simulink model "TV_Schema"  (R2024b)
settings: Solver=VariableStepAuto  StartTime=0.0  StopTime=3  RelTol=1e-3
model workspace (MAT data in the model file):
  Cyf = 60000
  Cyr = 60000
  Izz = 3000
  lf = 1.2
  lr = 1.5
  m = 1500
  tf = 0.65
  vx0 = 20
libraries: slpidlib x1
settings Model: Creator=junhyeongdoh  LastModifiedBy=junhyeongdoh

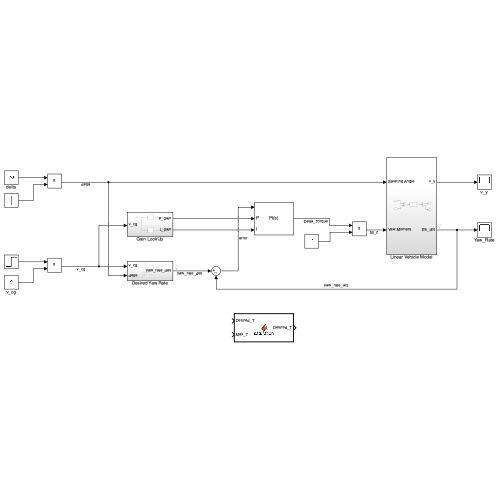
[thumbnail: Simulink's stored preview of the top-level diagram]
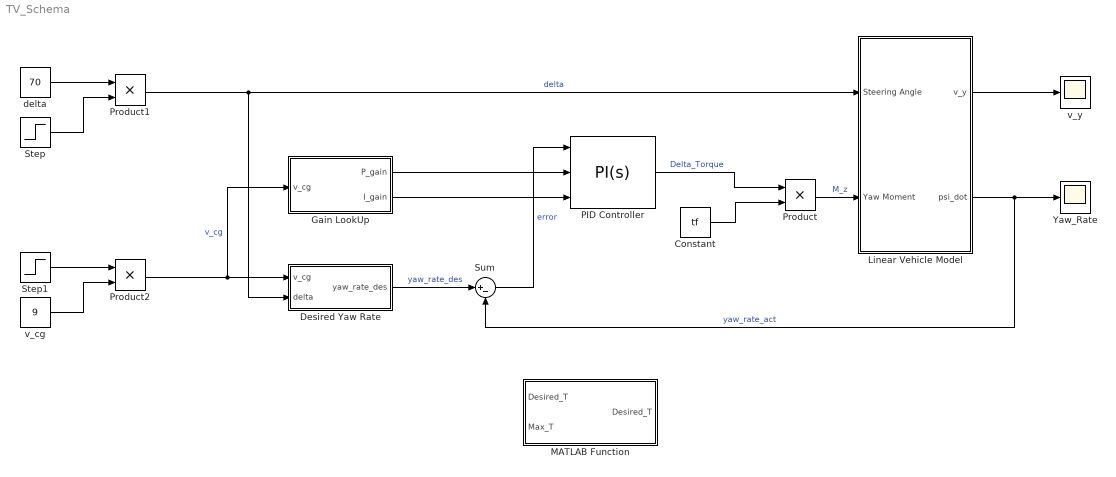
== system TV_Schema ==
  Constant : Constant  Value=tf
  Desired Yaw Rate : Subsystem
  Gain LookUp : Subsystem
  Linear Vehicle Model : Subsystem
  MATLAB Function : MATLAB Function  TreatAsAtomicUnit=on
  PID Controller : slpidlib/PID Controller  Controller=PI  Form=Parallel  TimeDomain=Continuous-time  UseExternalTs=off  SampleTime=-1  IntegratorMethod=Forward Euler  FilterMethod=Forward Euler  ControllerParametersSource=external  P=1  I=1  UseKiTs=off  D=0  UseExternalDerivativeSource=off  N=100  UseFilter=on  TunerSelectOption=Transfer Function Based (PID Tuner App)  InitialConditionSource=internal  InitialConditionForIntegrator=0  InitialConditionForFilter=0  DifferentiatorICPrevScaledInput=0  ExternalReset=none  TrackingMode=off  Kt=1  LimitOutput=off  SatLimitsSource=internal  UpperSaturationLimit=inf  LowerSaturationLimit=-inf  LinearizeAsGain=on  AntiWindupMode=none  Kb=1  LimitIntegrator=off  UpperIntegratorSaturationLimit=inf  LowerIntegratorSaturationLimit=-inf  POutMin=[]  POutMax=[]  IOutMin=[]  IOutMax=[]  DOutMin=[]  DOutMax=[]  NOutMin=[]  NOutMax=[]  SumOutMin=[]  SumOutMax=[]  SaturationOutMin=[]  SaturationOutMax=[]  PParamMin=[]  PParamMax=[]  IParamMin=[]  IParamMax=[]  DParamMin=[]  DParamMax=[]  NParamMin=[]  NParamMax=[]  KbParamMin=[]  KbParamMax=[]  KtParamMin=[]  KtParamMax=[]  KbOutMin=[]  KbOutMax=[]  KtOutMin=[]  KtOutMax=[]  IntegratorOutMin=[]  IntegratorOutMax=[]  FilterOutMin=[]  FilterOutMax=[]  SumI1OutMin=[]  SumI1OutMax=[]  SumI2OutMin=[]  SumI2OutMax=[]  SumI3OutMin=[]  SumI3OutMax=[]  SumI4OutMin=[]  SumI4OutMax=[]  SumDOutMin=[]  SumDOutMax=[]  DifferentiatorOutMin=[]  DifferentiatorOutMax=[]  FilterDiffOutCoefMin=[]  FilterDiffOutCoefMax=[]  ReciprocalOutMin=[]  ReciprocalOutMax=[]  SumDenOutMin=[]  SumDenOutMax=[]  SumNumOutMin=[]  SumNumOutMax=[]  DivideOutMin=[]  DivideOutMax=[]  UdiffTsProdOutMin=[]  UdiffTsProdOutMax=[]  NTsProdOutMin=[]  NTsProdOutMax=[]  UintegralTsProdOutMin=[]  UintegralTsProdOutMax=[]  UngainTsProdOutMin=[]  UngainTsProdOutMax=[]  ClampingZeroOutDataTypeStr=Inherit: Inherit via back propagation  ClampingZeroOutMin=[]  ClampingZeroOutMax=[]  FilterDenConstantOutDataTypeStr=Inherit: Inherit via back propagation  FilterDenConstantOutMin=[]  FilterDenConstantOutMax=[]  PCopyOutDataTypeStr=Inherit: Inherit via back propagation  PCopyOutMin=[]  PCopyOutMax=[]  NCopyOutDataTypeStr=Inherit: Inherit via back propagation  NCopyOutMin=[]  NCopyOutMax=[]  IntegratorContinuousStateAttributes=''  IntegratorStateMustResolveToSignalObject=off  IntegratorRTWStateStorageClass=Auto  FilterContinuousStateAttributes=''  FilterStateMustResolveToSignalObject=off  FilterRTWStateStorageClass=Auto  ParallelPVariant=ExternalParameters  IdealPVariant=Disabled  IVariant=ExternalParameters  DVariant=Disabled  IntegratorVariant=Continuous  SatVariant=Disabled  AWVariant=Passthrough  PCopyVariant=Disabled  TRVariant=Disabled  FdbkBlocksVariant=Forward  IdealPFdbkVariant=Disabled  SatFdbkVariant=Disabled  DerivativeFilterVariant=Disabled  NVariant=Disabled  NCopyVariant=Disabled_SignalSpec  FilterICVariant=Disabled  IntegratorICVariant=InternalICs  ExternalResetVariant=Disabled  TRSumVariant=Passthrough  SumFdbkVariant=Disabled  SumVariant=Sum_PI  TsampFilterVariant=InternalTs  TsampNgainVariant=Passthrough  TsampIntegralVariant=Disabled_SignalSpec  ExternalSaturationOutDataTypeStr=Inherit: Same as second input  DerivativeSourceVariant=Disabled  PreIntVariant=InternalPreInt
  Product : Product
  Product1 : Product
  Product2 : Product
  Step : Step  SampleTime=0
  Step1 : Step  SampleTime=0
  Sum : Sum  Inputs=|+-
  Yaw_Rate : Scope
  delta : Constant  Value=70
  v_cg : Constant  Value=9
  v_y : Scope
  wires:
  v_cg/1 -> Product2/2
  Gain LookUp/1(P_gain) -> PID Controller/2
  Gain LookUp/2(I_gain) -> PID Controller/3
  delta/1 -> Product1/1
  Linear Vehicle Model/2(psi_dot) -> Yaw_Rate/1, Sum/2  "yaw_rate_act"
  Desired Yaw Rate/1(yaw_rate_des) -> Sum/1  "yaw_rate_des"
  Sum/1 -> PID Controller/1  "error"
  PID Controller/1 -> Product/1  "Delta_Torque"
  Constant/1 -> Product/2
  Product/1 -> Linear Vehicle Model/2(Yaw Moment)  "M_z"
  Linear Vehicle Model/1(v_y) -> v_y/1
  Step/1 -> Product1/2
  Product1/1 -> Desired Yaw Rate/2(delta), Linear Vehicle Model/1(Steering Angle)  "delta"
  Step1/1 -> Product2/1
  Product2/1 -> Gain LookUp/1(v_cg), Desired Yaw Rate/1(v_cg)  "v_cg"

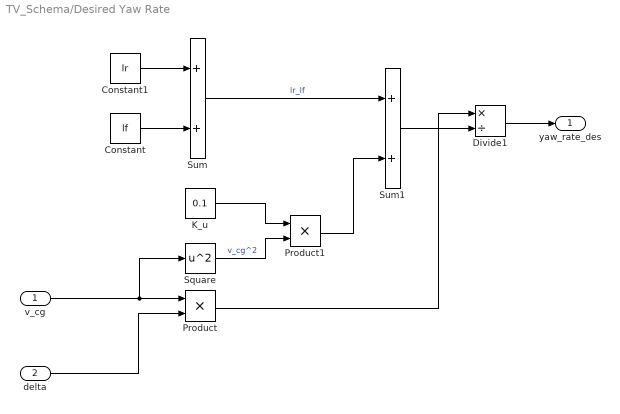
== system TV_Schema/Desired Yaw Rate ==
  v_cg : Inport
  delta : Inport  Port=2
  Constant : Constant  Value=lf
  Constant1 : Constant  Value=lr
  Divide1 : Product  Inputs=*/
  K_u : Constant  Value=0.1
  Product : Product
  Product1 : Product
  Square : Math  Operator=square
  Sum : Sum
  Sum1 : Sum
  yaw_rate_des : Outport
  wires:
  v_cg/1 -> Product/1, Square/1
  delta/1 -> Product/2
  Constant1/1 -> Sum/1
  Constant/1 -> Sum/2
  K_u/1 -> Product1/1
  Square/1 -> Product1/2  "v_cg^2"
  Sum/1 -> Sum1/1  "lr_lf"
  Product1/1 -> Sum1/2
  Sum1/1 -> Divide1/2
  Product/1 -> Divide1/1
  Divide1/1 -> yaw_rate_des/1

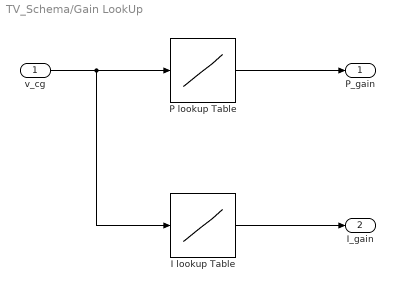
== system TV_Schema/Gain LookUp ==
  v_cg : Inport
  I lookup Table : Lookup_n-D  NumberOfTableDimensions=1  BreakpointsForDimension1=[7 10 13 16 19 22]  Table=[12716.7 12492.5 12040 11536.07 11058.5 13650]  InternalRulePriority=Speed  RndMeth=Simplest
  P lookup Table : Lookup_n-D  NumberOfTableDimensions=1  BreakpointsForDimension1=[7 10 13 16 19 22]  Table=[296.29 392.23 421.72 479.87 396.22 404.79]  InternalRulePriority=Speed  RndMeth=Simplest
  P_gain : Outport
  I_gain : Outport  Port=2
  wires:
  v_cg/1 -> I lookup Table/1, P lookup Table/1
  P lookup Table/1 -> P_gain/1
  I lookup Table/1 -> I_gain/1

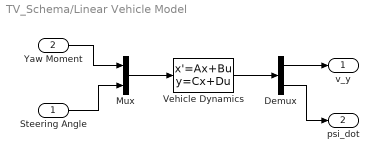
== system TV_Schema/Linear Vehicle Model ==
  Steering Angle : Inport
  Yaw Moment : Inport  Port=2
  Demux : Demux  Outputs=2
  Mux : Mux  Inputs=2
  Vehicle Dynamics : StateSpace  A=[-(Cyf + Cyr)/(m*vx0),(-lf*Cyf + lr*Cyr)/(m*vx0) - vx0; (-lf*Cyf + lr*Cyr)/(Izz*vx0),-(lf^2*Cyf + lr^2*Cyr)/(Izz*vx0)]  B=[[Cyf/(m*vx0); lf*Cyf/Izz], [0; 1/(0.05*Izz)]]  C=[1 0; 0 1]  D=[0 0; 0 0]  InitialCondition=[0; 0]
  v_y : Outport
  psi_dot : Outport  Port=2
  wires:
  Yaw Moment/1 -> Mux/1
  Demux/2 -> psi_dot/1
  Vehicle Dynamics/1 -> Demux/1
  Demux/1 -> v_y/1
  Mux/1 -> Vehicle Dynamics/1
  Steering Angle/1 -> Mux/2

== matlab function TV_Schema/MATLAB Function ==
  data: Desired_T output; Desired_T input; Max_T input
function Desired_T= saturation(Desired_T, Max_T)

if Desired_T > Max_T
    Desired_T = Max_T;
end
